simulink library "TargetPointing"  (R2014b)
settings: Solver=ode45  StartTime=0.0  StopTime=10.0  RelTol=1e-3
undefined symbols (not defined in the file or in its folder): confEstim, ConfParam
libraries: Normalization x3, Qprod x2, Mat2Quat x2, CrossProd x2, Qinverse x1, Quat2Rot x1, TransformMatrix x1, ECEFtoJ2000 x1
settings Model: Creator=Hp  LastModifiedBy=Hp

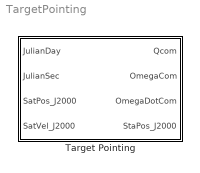
== system TargetPointing ==
  Target Pointing : Subsystem

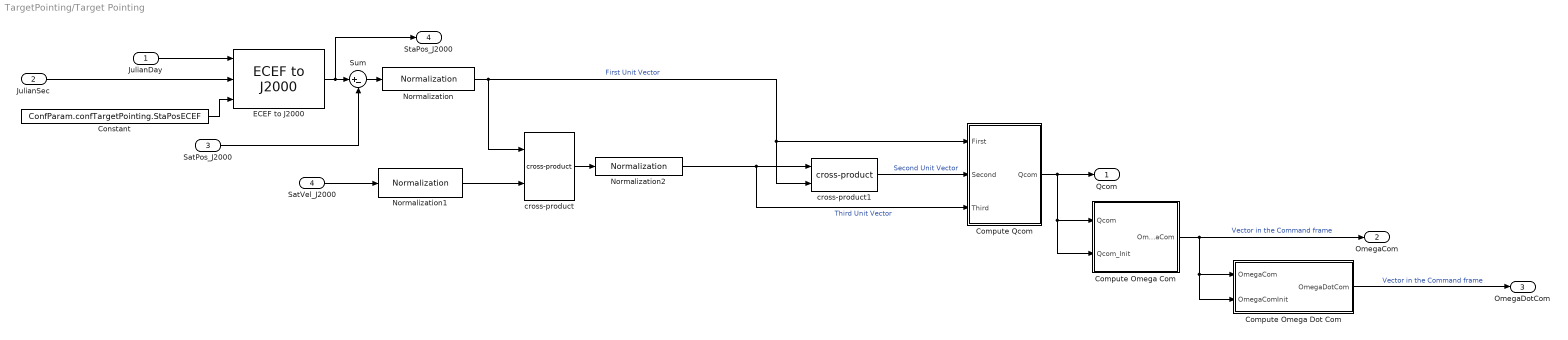
== system TargetPointing/Target Pointing ==
  JulianDay : Inport
  JulianSec : Inport  Port=2
  SatPos_J2000 : Inport  Port=3
  SatVel_J2000 : Inport  Port=4
  Compute Omega Com : Subsystem
  Compute Omega Dot Com : Subsystem
  Compute Qcom : Subsystem
  Constant : Constant  Value=ConfParam.confTargetPointing.StaPosECEF
  ECEF to J2000 : ECEFtoJ2000/ECEF to J2000
  Normalization : Normalization/Normalization
  Normalization1 : Normalization/Normalization
  Normalization2 : Normalization/Normalization
  Sum : Sum  Inputs=|+-
  cross-product : CrossProd/cross-product
  cross-product1 : CrossProd/cross-product
  Qcom : Outport
  OmegaCom : Outport  Port=2
  OmegaDotCom : Outport  Port=3
  StaPos_J2000 : Outport  Port=4
  wires:
  Sum/1 -> Normalization/1
  JulianSec/1 -> ECEF to J2000/2
  JulianDay/1 -> ECEF to J2000/1
  Constant/1 -> ECEF to J2000/3
  Compute Omega Dot Com/1(OmegaDotCom) -> OmegaDotCom/1  "Vector in the Command frame"
  Compute Omega Com/1(OmegaCom) -> OmegaCom/1, Compute Omega Dot Com/1(OmegaCom), Compute Omega Dot Com/2(OmegaComInit)  "Vector in the Command frame"
  SatPos_J2000/1 -> Sum/2
  cross-product/1 -> Normalization2/1
  SatVel_J2000/1 -> Normalization1/1
  ECEF to J2000/1 -> StaPos_J2000/1, Sum/1
  Normalization/1 -> cross-product/1, Compute Qcom/1(First), cross-product1/2  "First Unit Vector"
  Compute Qcom/1(Qcom) -> Qcom/1, Compute Omega Com/2(Qcom_Init), Compute Omega Com/1(Qcom)
  cross-product1/1 -> Compute Qcom/2(Second)  "Second Unit Vector"
  Normalization1/1 -> cross-product/2
  Normalization2/1 -> Compute Qcom/3(Third), cross-product1/1  "Third Unit Vector"

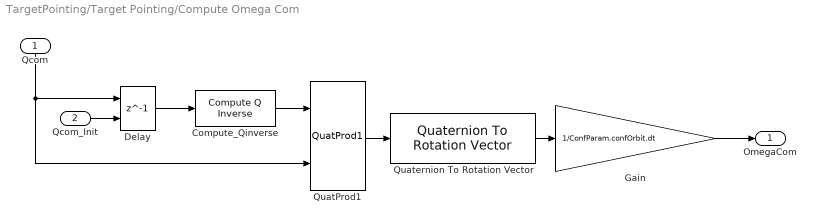
== system TargetPointing/Target Pointing/Compute Omega Com ==
  Qcom : Inport
  Qcom_Init : Inport  Port=2
  Compute_Qinverse : Qinverse/Compute Q Inverse
  Delay : Delay  DelayLength=1  InitialConditionSource=Input port  InitialCondition=confEstim.InitQsat  SampleTime=ConfParam.confOrbit.dt
      settings: InputPortMap=u0,p4
  Gain : Gain  Gain=1/ConfParam.confOrbit.dt
  QuatProd1 : Qprod/QuatProd1
  Quaternion To Rotation Vector : Quat2Rot/Quaternion To Rotation Vector
  OmegaCom : Outport
  wires:
  Qcom/1 -> QuatProd1/2, Delay/1
  Quaternion To Rotation Vector/1 -> Gain/1
  Gain/1 -> OmegaCom/1
  QuatProd1/1 -> Quaternion To Rotation Vector/1
  Delay/1 -> Compute_Qinverse/1
  Qcom_Init/1 -> Delay/2
  Compute_Qinverse/1 -> QuatProd1/1

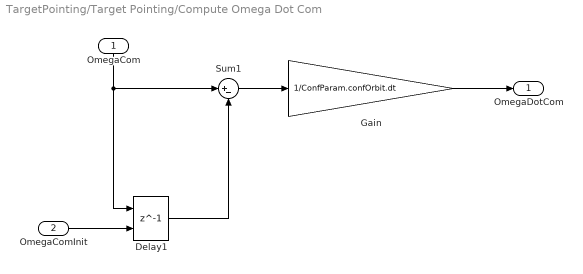
== system TargetPointing/Target Pointing/Compute Omega Dot Com ==
  OmegaCom : Inport
  OmegaComInit : Inport  Port=2
  Delay1 : Delay  DelayLength=1  InitialConditionSource=Input port  InitialCondition=confEstim.InitQsat  SampleTime=ConfParam.confOrbit.dt
      settings: InputPortMap=u0,p4
  Gain : Gain  Gain=1/ConfParam.confOrbit.dt
  Sum1 : Sum  Inputs=|+-
  OmegaDotCom : Outport
  wires:
  OmegaCom/1 -> Sum1/1, Delay1/1
  Gain/1 -> OmegaDotCom/1
  Sum1/1 -> Gain/1
  OmegaComInit/1 -> Delay1/2
  Delay1/1 -> Sum1/2

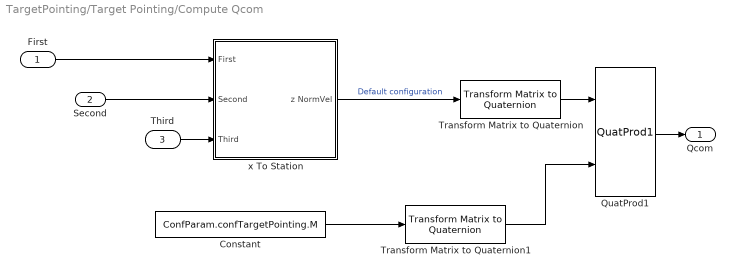
== system TargetPointing/Target Pointing/Compute Qcom ==
  First : Inport
  Second : Inport  Port=2
  Third : Inport  Port=3
  Constant : Constant  Value=ConfParam.confTargetPointing.M
  QuatProd1 : Qprod/QuatProd1
  Transform Matrix to Quaternion : Mat2Quat/Transform Matrix to Quaternion
  Transform Matrix to Quaternion1 : Mat2Quat/Transform Matrix to Quaternion
  x To Station : Subsystem
  Qcom : Outport
  wires:
  Transform Matrix to Quaternion/1 -> QuatProd1/1
  Third/1 -> x To Station/3(Third)
  Second/1 -> x To Station/2(Second)
  First/1 -> x To Station/1(First)
  x To Station/1(z NormVel) -> Transform Matrix to Quaternion/1  "Default configuration"
  Transform Matrix to Quaternion1/1 -> QuatProd1/2
  QuatProd1/1 -> Qcom/1
  Constant/1 -> Transform Matrix to Quaternion1/1

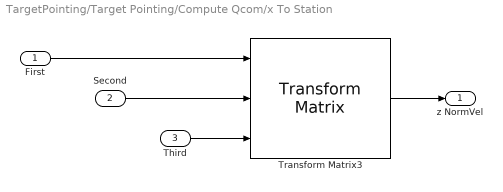
== system TargetPointing/Target Pointing/Compute Qcom/x To Station ==
  First : Inport
  Second : Inport  Port=2
  Third : Inport  Port=3
  Transform Matrix3 : TransformMatrix/Transform Matrix
  z NormVel : Outport
  wires:
  Transform Matrix3/1 -> z NormVel/1
  Second/1 -> Transform Matrix3/2
  First/1 -> Transform Matrix3/1
  Third/1 -> Transform Matrix3/3
